simulink model "chap14_2sim"  (Simulink 7.7)
settings: Solver=ode45  StartTime=0.0  StopTime=10.0  RelTol=1e-3
settings Model: Creator=liujk  LastModifiedBy=ljk
settings DataIOCC: SignalLoggingName=sigsOut
settings OptimizationCC: ExpressionDepthLimit=128
settings DebuggingCC: SaveWithParameterizedLinksMsg=none  SignalResolutionControl=TryResolveAllWithWarning  SolverPrmCheckMsg=none  MultiTaskDSMMsg=warning  MultiTaskCondExecSysMsg=none  StrictBusMsg=None
settings HardwareCC: TargetUnknown=on
settings RTWCC: IncludeERTFirstTime=on
settings CodeAppCC: CustomSymbolStrType=$N$R$M_T

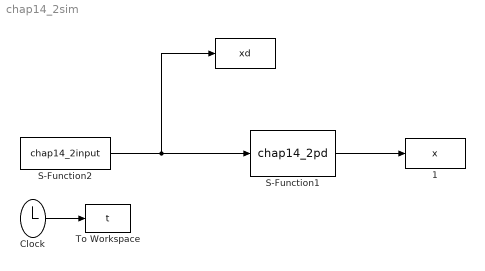
== system chap14_2sim ==
  "  " : ToWorkspace  VariableName=xd  SampleTime=-1  SaveFormat=Array
  "  1" : ToWorkspace  VariableName=x  SampleTime=-1  SaveFormat=Array
  Clock : Clock
      settings: Decimation=10
  S-Function1 : S-Function  FunctionName=chap14_2pd  EnableBusSupport=off
  S-Function2 : S-Function  FunctionName=chap14_2input  EnableBusSupport=off
  To Workspace : ToWorkspace  VariableName=t  SampleTime=-1  SaveFormat=Array
  wires:
  S-Function1/1 -> "  1"/1
  Clock/1 -> To Workspace/1
  S-Function2/1 -> "  "/1, S-Function1/1
